simulink model "cmde_robot_mod"  (R2013a)
settings: Solver=ode45  StartTime=0.0  StopTime=10  FixedStep=0.005  RelTol=1e-3
values from neighbouring files (symbols this model uses):
  B1 = a1 + a2*cq2    [mgi_mitsu.m]
undefined symbols (not defined in the file or in its folder): A1, B, Jeff1, Jeff2, Km, Kmat1, Kp1, qConsigne1, qInitial, R, r
settings Model: Creator=Mylene  LastModifiedBy=user
settings DataIOCC: SignalLoggingSaveFormat=ModelDataLogs
settings OptimizationCC: ExpressionDepthLimit=2147483647
settings DebuggingCC: FcnCallInpInsideContextMsg=UseLocalSettings
settings GRTTargetCC: CombineOutputUpdateFcns=off  GRTInterface=on

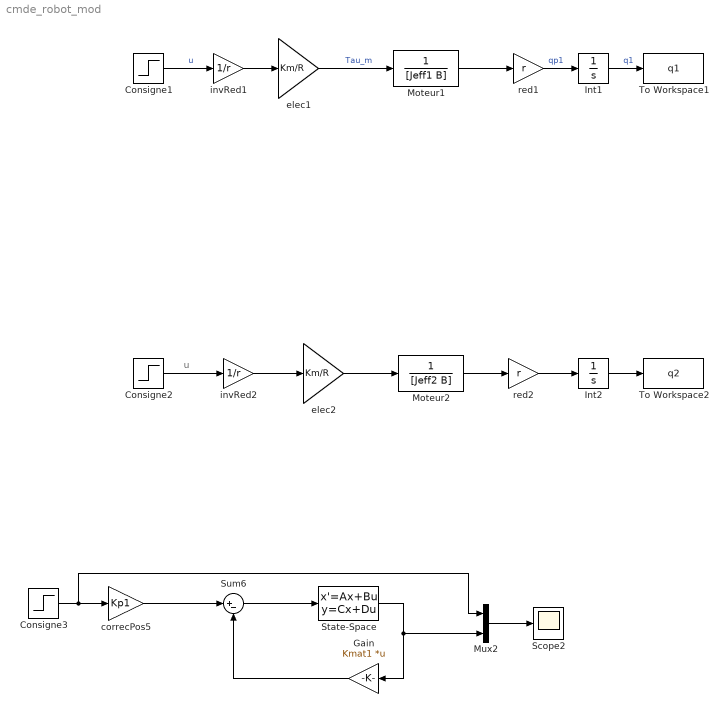
== system cmde_robot_mod ==
  note: u
  Consigne1 : Step  SampleTime=1
  Consigne2 : Step  SampleTime=0
  Consigne3 : Step  Before=qInitial  After=qConsigne1  SampleTime=0
  Gain : Gain  Gain=Kmat1  Multiplication=Matrix(K*u)
  Int1 : Integrator  InitialCondition=qInitial
  Int2 : Integrator  InitialCondition=qInitial
  Moteur1 : TransferFcn  Denominator=[Jeff1 B]
  Moteur2 : TransferFcn  Denominator=[Jeff2 B]
  Mux2 : Mux  Inputs=2
  Scope2 : Scope
      settings: TimeRange=10  YMin=0  YMax=0.8  SaveName=ScopeData2
  State-Space : StateSpace  A=A1  B=B1  C=eye(2)  D=zeros(2,1)
  Sum6 : Sum  Inputs=|+-
  To Workspace1 : ToWorkspace  VariableName=q1  SampleTime=-1
  To Workspace2 : ToWorkspace  VariableName=q2  SampleTime=-1
  correcPos5 : Gain  Gain=Kp1
  elec1 : Gain  Gain=Km/R
  elec2 : Gain  Gain=Km/R
  invRed1 : Gain  Gain=1/r
  invRed2 : Gain  Gain=1/r
  red1 : Gain  Gain=r
  red2 : Gain  Gain=r
  wires:
  elec1/1 -> Moteur1/1  "Tau_m"
  elec2/1 -> Moteur2/1
  Consigne2/1 -> invRed2/1
  red1/1 -> Int1/1  "qp1"
  Moteur1/1 -> red1/1
  Int1/1 -> To Workspace1/1  "q1"
  Moteur2/1 -> red2/1
  red2/1 -> Int2/1
  Int2/1 -> To Workspace2/1
  invRed1/1 -> elec1/1
  Consigne1/1 -> invRed1/1  "u"
  invRed2/1 -> elec2/1
  Consigne3/1 -> correcPos5/1, Mux2/1
  Sum6/1 -> State-Space/1
  State-Space/1 -> Gain/1, Mux2/2
  Gain/1 -> Sum6/2
  Mux2/1 -> Scope2/1
  correcPos5/1 -> Sum6/1
